simulink model "testing_differential"  (R2015a)
settings: Solver=ode45  StartTime=0.0  StopTime=inf  FixedStep=0.001  RelTol=1e-3
values from neighbouring files (symbols this model uses):
  colors = [colors;colors_rotor]    [sketch_copter.m]
  F = thrust_c    [attitude_controller.m]    (also in quad_dynamics.m = uu(1); sketch_copter.m = [F;F_rotor+rotor*size(V_rotor,1)]; testing_dynamics.m = uu(1))
  forces_moments = [fz; l; m; n]    [forces_moments.m]
  V = V*R    [drawAircraft.m]    (also in sketch_copter.m = [V;V_rotor*R]; testing_drawAircraft.m)
undefined symbols (not defined in the file or in its folder): attitude_controller, P, testing_diff, testing_drawAircraft, testing_inverse, trajectory
settings Model: NumberOfSteps=100  Creator=ecestudent  LastModifiedBy=ecestudent

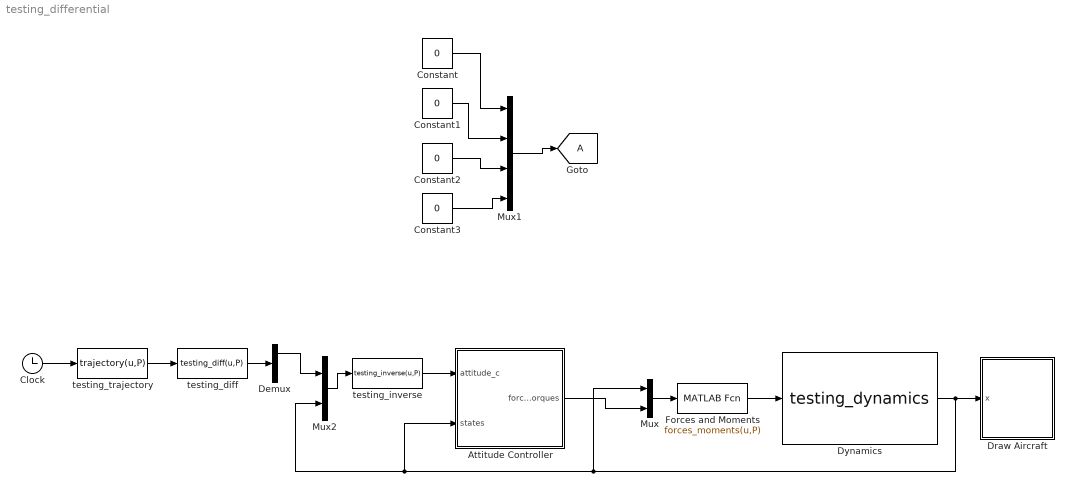
== system testing_differential ==
  Attitude Controller : Subsystem
      mask Display: image(imread('images/auto_pilot.jpg'))
  Clock : Clock
  Constant{,1..3} (4 alike) : Constant  Value=0
  Demux : Demux  Outputs=[4 7]
  Draw Aircraft : Subsystem
      mask Display: image(imread('images/tv.jpg'))
  Dynamics : S-Function  FunctionName=testing_dynamics  Parameters=P
      mask Display: image(imread('images/hexacopter.png'))
  Forces and Moments : MATLABFcn  MATLABFcn=forces_moments(u,P)  OutputDimensions=4
  Mux : Mux  Inputs=2
  Mux1 : Mux
  Mux2 : Mux  Inputs=2
  testing_diff : MATLABFcn  MATLABFcn=testing_diff(u,P)  OutputDimensions=11
  testing_inverse : MATLABFcn  MATLABFcn=testing_inverse(u,P)  OutputDimensions=4
  testing_trajectory : MATLABFcn  MATLABFcn=trajectory(u,P)  OutputDimensions=11
  tag scope: A=global
  wires:
  Mux/1 -> Forces and Moments/1
  Attitude Controller/1(force_torques) -> Mux/2
  Dynamics/1 -> Draw Aircraft/1(x), Attitude Controller/2(states), Mux2/2, Mux/1
  Forces and Moments/1 -> Dynamics/1
  testing_inverse/1 -> Attitude Controller/1(attitude_c)
  Constant/1 -> Mux1/1
  Constant1/1 -> Mux1/2
  Constant2/1 -> Mux1/3
  Constant3/1 -> Mux1/4
  Mux1/1 -> [A]
  Mux2/1 -> testing_inverse/1
  testing_trajectory/1 -> testing_diff/1
  testing_diff/1 -> Demux/1
  Demux/1 -> Mux2/1
  Clock/1 -> testing_trajectory/1

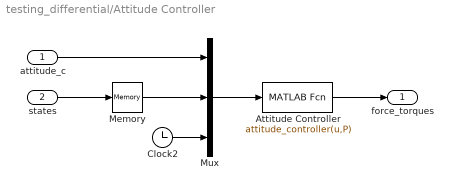
== system testing_differential/Attitude Controller ==
  attitude_c : Inport
  states : Inport  Port=2
  Attitude Controller : MATLABFcn  MATLABFcn=attitude_controller(u,P)  OutputDimensions=4  SampleTime=0.002
  Clock2 : Clock
  Memory : Memory
  Mux : Mux  Inputs=3
  force_torques : Outport
  wires:
  Clock2/1 -> Mux/3
  Mux/1 -> Attitude Controller/1
  Attitude Controller/1 -> force_torques/1
  states/1 -> Memory/1
  Memory/1 -> Mux/2
  attitude_c/1 -> Mux/1

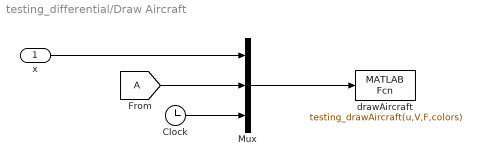
== system testing_differential/Draw Aircraft ==
  x : Inport
  Clock : Clock
  Mux : Mux  Inputs=3
  drawAircraft : MATLABFcn  MATLABFcn=testing_drawAircraft(u,V,F,colors)  OutputDimensions=0  SampleTime=0.1
  wires:
  x/1 -> Mux/1
  [A] -> Mux/2
  Mux/1 -> drawAircraft/1
  Clock/1 -> Mux/3
